simulink model "rudder_response"  (Simulink 6.6)
settings: Solver=ode3  StartTime=0.0  StopTime=5  FixedStep=T_step  RelTol=1e-3
undefined symbols (not defined in the file or in its folder): damping_rudder, I_rudder, K_d_rudder, K_i_rudder, K_p_rudder, stiffness_rudder
settings Model: Creator=Administrator  LastModifiedBy=Administrator

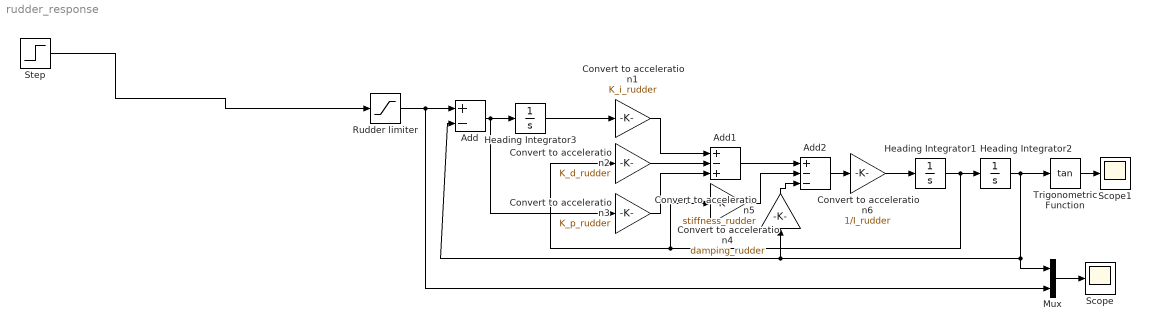
== system rudder_response ==
  Add : Sum  Inputs=+-  OutScaling=2^-10
  Add1 : Sum  Inputs=+-+  OutScaling=2^-10
  Add2 : Sum  Inputs=+--  OutScaling=2^-10
  Convert to acceleration1 : Gain  Gain=K_i_rudder
  Convert to acceleration2 : Gain  Gain=K_d_rudder
  Convert to acceleration3 : Gain  Gain=K_p_rudder
  Convert to acceleration4 : Gain  Gain=damping_rudder
  Convert to acceleration5 : Gain  Orientation=up  Gain=stiffness_rudder
  Convert to acceleration6 : Gain  Gain=1/I_rudder
  Heading Integrator1 : Integrator  LimitOutput=on  UpperSaturationLimit=10  LowerSaturationLimit=-10
  Heading Integrator2 : Integrator  LimitOutput=on  UpperSaturationLimit=1  LowerSaturationLimit=-1
  Heading Integrator3 : Integrator  LimitOutput=on  UpperSaturationLimit=10  LowerSaturationLimit=-10
  Mux : Mux  Inputs=2
  Rudder limiter : Saturate  UpperLimit=1  LowerLimit=-1
  Scope : Scope
      settings: YMin=0.95  YMax=1.05
  Scope1 : Scope
  Step : Step  Before=1  After=0
  Trigonometric Function : Trigonometry  Operator=tan  OutputSignalType=real
  wires:
  Rudder limiter/1 -> Add/1, Mux/2
  Add/1 -> Convert to acceleration3/1, Heading Integrator3/1
  Convert to acceleration1/1 -> Add1/1
  Convert to acceleration2/1 -> Add1/2
  Heading Integrator1/1 -> Heading Integrator2/1, Convert to acceleration2/1, Convert to acceleration4/1
  Heading Integrator2/1 -> Convert to acceleration5/1, Add/2, Mux/1, Trigonometric Function/1
  Convert to acceleration3/1 -> Add1/3
  Add1/1 -> Add2/1
  Convert to acceleration4/1 -> Add2/2
  Convert to acceleration5/1 -> Add2/3
  Add2/1 -> Convert to acceleration6/1
  Convert to acceleration6/1 -> Heading Integrator1/1
  Heading Integrator3/1 -> Convert to acceleration1/1
  Mux/1 -> Scope/1
  Step/1 -> Rudder limiter/1
  Trigonometric Function/1 -> Scope1/1
